simulink model "plant2"  (Simulink 9.3)
settings: Solver=VariableStepAuto  StartTime=0.0  StopTime=10.0  RelTol=1e-3
settings Model: Creator=Lenovo  LastModifiedBy=Lenovo
settings DataIOCC: SaveFormat=Dataset  SignalLoggingSaveFormat=Dataset
settings OptimizationCC: LifeSpan=auto
settings DebuggingCC: UnderspecifiedInitializationDetection=Simplified  MergeDetectMultiDrivingBlocksExec=error  FcnCallInpInsideContextMsg=error  SFUnexpectedBacktrackingDiag=error  SFNoUnconditionalDefaultTransitionDiag=error  SFExecutionAtInitializationDiag=warning  ArithmeticOperatorsInVariantConditions=error
settings HardwareCC: ProdBitPerPointer=64  ProdBitPerSizeT=64  ProdBitPerPtrDiffT=64  ProdLargestAtomicFloat=Float  ProdIntDivRoundTo=Zero  ProdEndianess=LittleEndian  ProdWordSize=64  ProdHWDeviceType=Intel->x86-64 (Windows64)
settings ModelReferenceCC: PropagateSignalLabelsOutOfModel=on
settings SFSimCC: SimUseLocalCustomCode=on
settings RTWCC: RTWUseLocalCustomCode=on
settings CodeAppCC: StateflowObjectComments=off
settings GRTTargetCC: TargetLangStandard=C99 (ISO)  CombineOutputUpdateFcns=on  GRTInterface=off
settings ConfigComp: CovMetricSettings=dwe  CovHtmlReporting=off  CovSaveCumulativeToWorkspaceVar=off  CovSaveSingleToWorkspaceVar=off  CovExternalEMLEnable=on

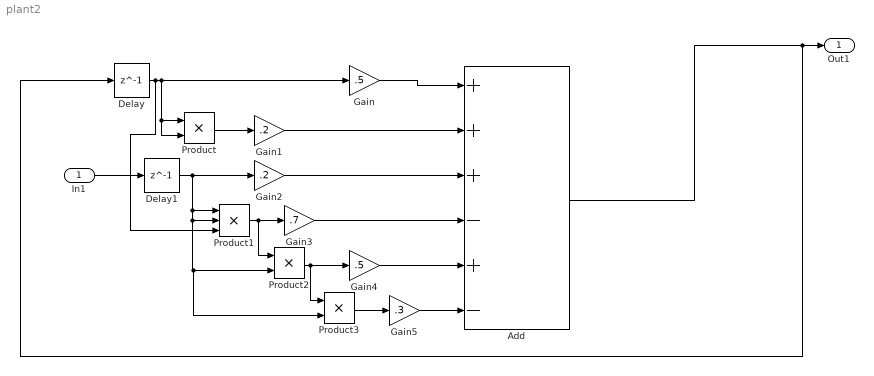
== system plant2 ==
  In1 : Inport
  Add : Sum  Inputs=+++-+-
  Delay : Delay  DelayLength=1  InitialCondition=0
  Delay1 : Delay  DelayLength=1  InitialCondition=0
  Gain : Gain  Gain=.5
  Gain1 : Gain  Gain=.2
  Gain2 : Gain  Gain=.2
  Gain3 : Gain  Gain=.7
  Gain4 : Gain  Gain=.5
  Gain5 : Gain  Gain=.3
  Product : Product
  Product1 : Product  Inputs=3
  Product2 : Product
  Product3 : Product
  Out1 : Outport
  wires:
  In1/1 -> Delay1/1
  Delay/1 -> Product1/3, Product/2, Product/1, Gain/1
  Gain5/1 -> Add/6
  Gain2/1 -> Add/3
  Product3/1 -> Gain5/1
  Add/1 -> Out1/1, Delay/1
  Gain4/1 -> Add/5
  Product2/1 -> Product3/1, Gain4/1
  Delay1/1 -> Product3/2, Product2/2, Product1/2, Product1/1, Gain2/1
  Gain3/1 -> Add/4
  Product1/1 -> Product2/1, Gain3/1
  Product/1 -> Gain1/1
  Gain1/1 -> Add/2
  Gain/1 -> Add/1
